simulink model "W01_Base_Map_cs"  (R2019a)
settings: Solver=FixedStepDiscrete  StartTime=0.0  StopTime=40  FixedStep=1/20  RelTol=1e-3
PreLoadFcn:
  | mbxruntime.callbacks.PreLoadFcn(bdroot);
  | check_NUTS_defined
  | model_closed = 0;
  | assignin('base',['model_closed_' bdroot],false);
PostLoadFcn:
  | mbxruntime.callbacks.PostLoadFcn(bdroot);
InitFcn:
  | mbxruntime.callbacks.InitFcn(bdroot);
StartFcn:
  | mbxruntime.callbacks.StartFcn(bdroot);
StopFcn:
  | mbxruntime.callbacks.StopFcn(bdroot);;
  | 
model workspace: external: MAT-File .\W01_Base_Map_cs_hws.mat (data not in the file)
undefined symbols (not defined in the file or in its folder): DiscIntNeverNeededParam, InitImageOutputDir, mbxruntime, tabledata, W01_Base_Map_cs_328ec7e3a8cd5b54, W01_Base_Map_cs_423c72fa17799c7f, W01_Base_Map_cs_514c2dea2cdbe680, W01_Base_Map_cs_51d6e6e467bedba1, W01_Base_Map_cs_563ebd29d1fd6c09, W01_Base_Map_cs_57ea59d0358dab77, W01_Base_Map_cs_669d1acb174df2b9, W01_Base_Map_cs_774a522413284ef7, W01_Base_Map_cs_9538d35a279fbe4e, W01_Base_Map_cs_9f504bb84aebc2fd, W01_Base_Map_cs_a242ed7539861165, W01_Base_Map_cs_ae41b72d7e14f81d, W01_Base_Map_cs_Audi_A8_Sedan_1_Path_pathUniqueID, W01_Base_Map_cs_b5931a786e299506, W01_Base_Map_cs_b7f45a070fa6e639, W01_Base_Map_cs_c02beb48492dde12, W01_Base_Map_cs_c75b75e9f6b035bf, W01_Base_Map_cs_cf83ac8e8b053cbf, W01_Base_Map_cs_Child_RegularAni_1_Path_pathUniqueID, W01_Base_Map_cs_Child_RegularAni_2_Path_pathUniqueID, W01_Base_Map_cs_Citroen_C3_Hatchback_1_Path_pathUniqueID, W01_Base_Map_cs_d4423fcf1c0d6fc4, W01_Base_Map_cs_df133aa86d9852fe, W01_Base_Map_cs_Female_RegularAni_1_Path_pathUniqueID, W01_Base_Map_cs_Male_RegularAni_1_Path_pathUniqueID, W01_Base_Map_cs_Male_RegularAni_2_Path_pathUniqueID
libraries: simulink_extras x41, adeye_lib x15, simulink x10, dspindex x6, PreScanSimulinkLibrary x4, sharedtransform x3, robotcorelib x1, PreScanUsefulBlocks x1
(part 8 of 11)

== system W01_Base_Map_cs/BMW_X5_SUV_1/PointCloudSensor_4_Angles_Demux ==
  In2 : Inport
  Selector : Selector  NumberOfDimensions=2  InputPortWidth=3  IndexOptions=Index vector (dialog),Index vector (dialog)  Indices=-1,offset+1:(offset+hres)  OutputSizes=1,1
  Selector1 : Selector  NumberOfDimensions=2  InputPortWidth=3  IndexOptions=Index vector (dialog),Index vector (dialog)  Indices=-1,(offset+hres+1):(offset+2*hres)  OutputSizes=1,1
  Theta : Outport
  Phi : Outport  Port=2
  wires:
  Selector1/1 -> Phi/1
  Selector/1 -> Theta/1
  In2/1 -> Selector/1, Selector1/1

== system W01_Base_Map_cs/BMW_X5_SUV_1/PointCloudSensor_4_Intensity_Demux ==
  In1 : Inport
  Selector3 : Selector  NumberOfDimensions=2  InputPortWidth=3  IndexOptions=Index vector (dialog),Index vector (dialog)  Indices=-1,offset+1:(offset+hres)  OutputSizes=1,1
  Intensity : Outport
  wires:
  Selector3/1 -> Intensity/1
  In1/1 -> Selector3/1

== system W01_Base_Map_cs/BMW_X5_SUV_1/PointCloudSensor_4_Range_Demux ==
  In1 : Inport
  Selector : Selector  NumberOfDimensions=2  InputPortWidth=3  IndexOptions=Index vector (dialog),Index vector (dialog)  Indices=-1,offset+1:(offset+hres)  OutputSizes=1,1
  Range : Outport
  wires:
  Selector/1 -> Range/1
  In1/1 -> Selector/1

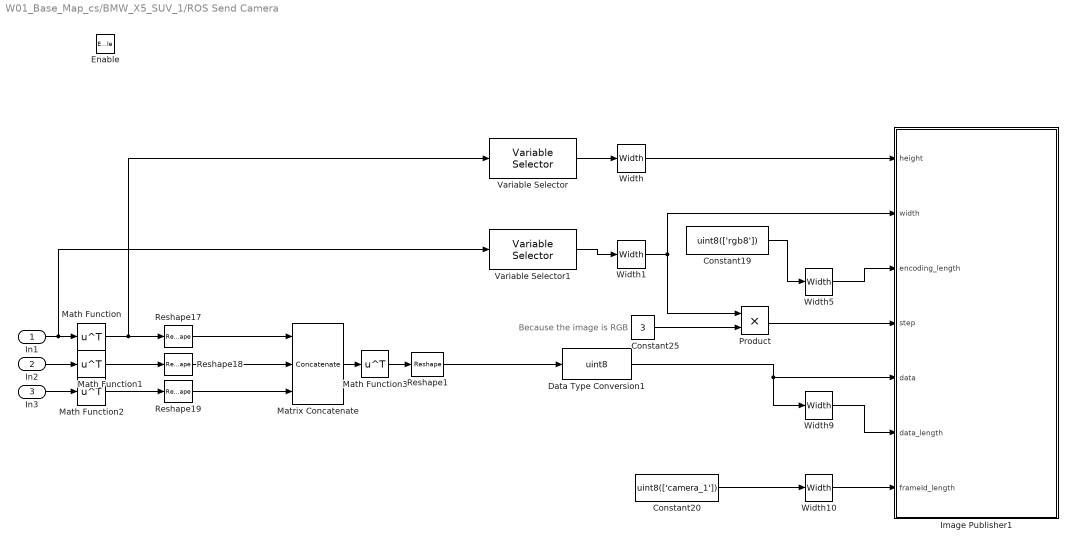
== system W01_Base_Map_cs/BMW_X5_SUV_1/ROS Send Camera ==
  note: Because the image is RGB
  In1 : Inport
  In2 : Inport  Port=2
  In3 : Inport  Port=3
  Enable : EnablePort
  Constant19 : Constant  Value=uint8(['rgb8'])
  Constant20 : Constant  Value=uint8(['camera_1'])
  Constant25 : Constant  Value=3  OutDataTypeStr=Inherit: Inherit via back propagation
  Data Type Conversion1 : DataTypeConversion  OutDataTypeStr=uint8
  Image Publisher1 : Subsystem  mask{topic='/camera_1/image_raw', message_type='sensor_msgs/Image', port=9090, timeout=2, frame_id='camera_1'}
      mask prompts: topic "Topic name"; message_type "Message type"; timeout "Timeout (s)"; frame_id "Frame id (keep '/default' if it's not used)"
  Math Function{,1..3} (4 alike) : Math  Operator=transpose  SaturateOnIntegerOverflow=on
  Matrix Concatenate : Concatenate  NumInputs=3  Mode=Multidimensional array  ConcatenateDimension=2
  Product : Product  OutDataTypeStr=uint32
  Reshape{1,17..19} (4 alike) : Reshape
  Variable Selector : dspindex/Variable Selector  NumInputs=1  rowsOrCols=Rows  IdxMode=Fixed  Elements=[1]  ZerOneIdxMode=One-based  errmode=Clip Index  FillMode=on  FillValues=0
  Variable Selector1 : dspindex/Variable Selector  NumInputs=1  rowsOrCols=Rows  IdxMode=Fixed  Elements=[1]  ZerOneIdxMode=One-based  errmode=Clip Index  FillMode=on  FillValues=0
  Width : Width
  Width1 : Width
  Width10 : Width  DataType=uint32
  Width5 : Width  DataType=uint32
  Width9 : Width  DataType=uint32
  wires:
  Math Function3/1 -> Reshape1/1
  Matrix Concatenate/1 -> Math Function3/1
  In1/1 -> Variable Selector1/1, Math Function/1
  In2/1 -> Math Function1/1
  In3/1 -> Math Function2/1
  Math Function1/1 -> Reshape18/1
  Math Function2/1 -> Reshape19/1
  Reshape17/1 -> Matrix Concatenate/1
  Reshape18/1 -> Matrix Concatenate/2
  Math Function/1 -> Variable Selector/1, Reshape17/1
  Reshape19/1 -> Matrix Concatenate/3
  Constant20/1 -> Width10/1
  Constant25/1 -> Product/2
  Variable Selector1/1 -> Width1/1
  Data Type Conversion1/1 -> Image Publisher1/5(data), Width9/1
  Constant19/1 -> Width5/1
  Variable Selector/1 -> Width/1
  Width1/1 -> Image Publisher1/2(width), Product/1
  Reshape1/1 -> Data Type Conversion1/1
  Width/1 -> Image Publisher1/1(height)
  Product/1 -> Image Publisher1/4(step)
  Width10/1 -> Image Publisher1/7(frameId_length)
  Width5/1 -> Image Publisher1/3(encoding_length)
  Width9/1 -> Image Publisher1/6(data_length)

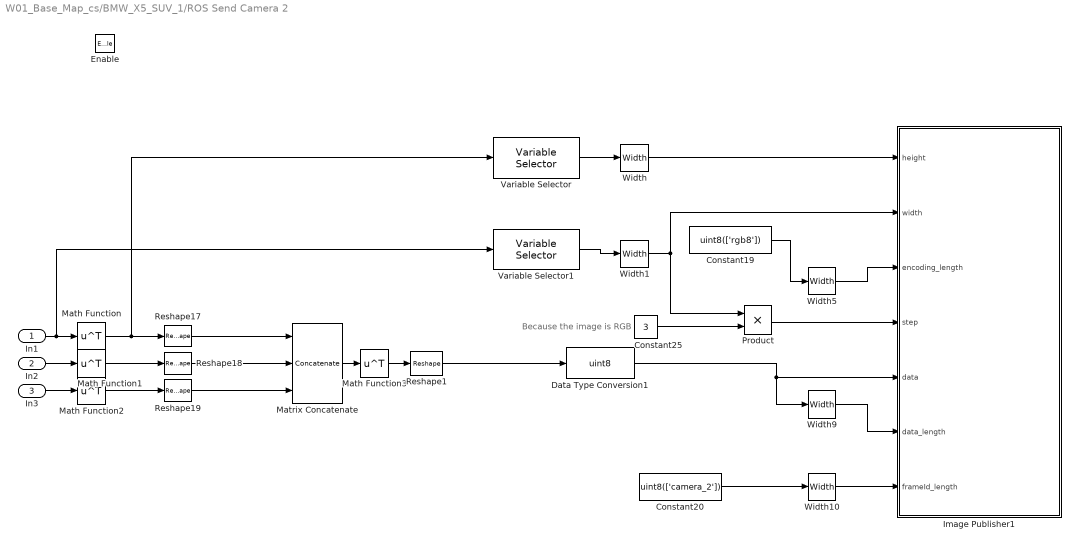
== system W01_Base_Map_cs/BMW_X5_SUV_1/ROS Send Camera 2 ==
  note: Because the image is RGB
  In1 : Inport
  In2 : Inport  Port=2
  In3 : Inport  Port=3
  Enable : EnablePort
  Constant19 : Constant  Value=uint8(['rgb8'])
  Constant20 : Constant  Value=uint8(['camera_2'])
  Constant25 : Constant  Value=3  OutDataTypeStr=Inherit: Inherit via back propagation
  Data Type Conversion1 : DataTypeConversion  OutDataTypeStr=uint8
  Image Publisher1 : Subsystem  mask{topic='/camera_2/image_raw', message_type='sensor_msgs/Image', port=9090, timeout=2, frame_id='camera_2'}
      mask prompts: topic "Topic name"; message_type "Message type"; timeout "Timeout (s)"; frame_id "Frame id (keep '/default' if it's not used)"
  Math Function{,1..3} (4 alike) : Math  Operator=transpose  SaturateOnIntegerOverflow=on
  Matrix Concatenate : Concatenate  NumInputs=3  Mode=Multidimensional array  ConcatenateDimension=2
  Product : Product  OutDataTypeStr=uint32
  Reshape{1,17..19} (4 alike) : Reshape
  Variable Selector : dspindex/Variable Selector  NumInputs=1  rowsOrCols=Rows  IdxMode=Fixed  Elements=[1]  ZerOneIdxMode=One-based  errmode=Clip Index  FillMode=on  FillValues=0
  Variable Selector1 : dspindex/Variable Selector  NumInputs=1  rowsOrCols=Rows  IdxMode=Fixed  Elements=[1]  ZerOneIdxMode=One-based  errmode=Clip Index  FillMode=on  FillValues=0
  Width : Width
  Width1 : Width
  Width10 : Width  DataType=uint32
  Width5 : Width  DataType=uint32
  Width9 : Width  DataType=uint32
  wires:
  Math Function3/1 -> Reshape1/1
  Matrix Concatenate/1 -> Math Function3/1
  In1/1 -> Variable Selector1/1, Math Function/1
  In2/1 -> Math Function1/1
  In3/1 -> Math Function2/1
  Math Function1/1 -> Reshape18/1
  Math Function2/1 -> Reshape19/1
  Reshape17/1 -> Matrix Concatenate/1
  Reshape18/1 -> Matrix Concatenate/2
  Math Function/1 -> Variable Selector/1, Reshape17/1
  Reshape19/1 -> Matrix Concatenate/3
  Width1/1 -> Image Publisher1/2(width), Product/1
  Product/1 -> Image Publisher1/4(step)
  Variable Selector/1 -> Width/1
  Width/1 -> Image Publisher1/1(height)
  Width10/1 -> Image Publisher1/7(frameId_length)
  Data Type Conversion1/1 -> Image Publisher1/5(data), Width9/1
  Reshape1/1 -> Data Type Conversion1/1
  Constant20/1 -> Width10/1
  Variable Selector1/1 -> Width1/1
  Constant25/1 -> Product/2
  Width5/1 -> Image Publisher1/3(encoding_length)
  Width9/1 -> Image Publisher1/6(data_length)
  Constant19/1 -> Width5/1

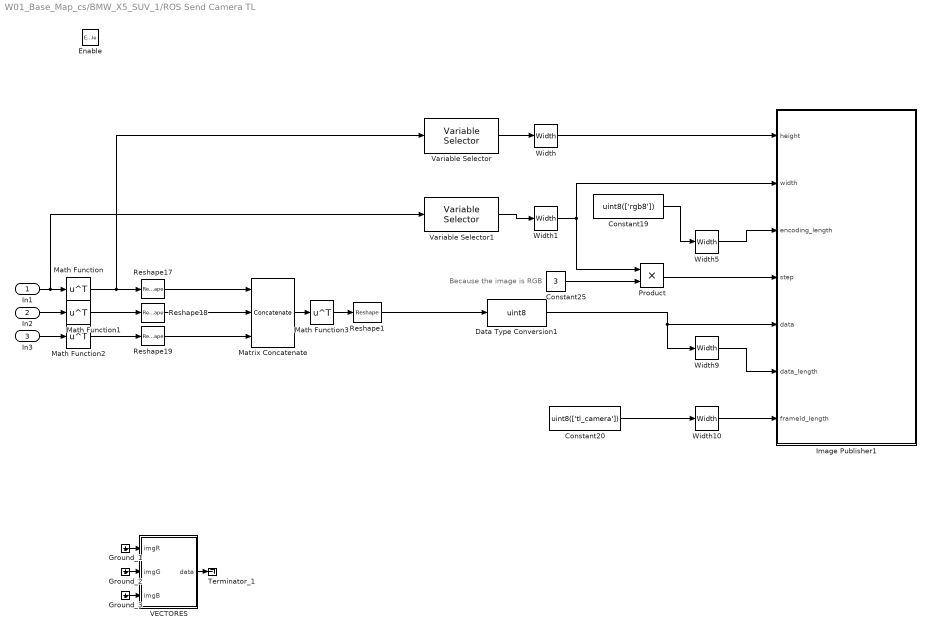
== system W01_Base_Map_cs/BMW_X5_SUV_1/ROS Send Camera TL ==
  note: Because the image is RGB
  In1 : Inport
  In2 : Inport  Port=2
  In3 : Inport  Port=3
  Enable : EnablePort
  Constant19 : Constant  Value=uint8(['rgb8'])
  Constant20 : Constant  Value=uint8(['tl_camera'])
  Constant25 : Constant  Value=3  OutDataTypeStr=Inherit: Inherit via back propagation
  Data Type Conversion1 : DataTypeConversion  OutDataTypeStr=uint8
  Ground_1 : Ground
  Ground_2 : Ground
  Ground_3 : Ground
  Image Publisher1 : Subsystem  mask{topic='/tl/image_raw', message_type='sensor_msgs/Image', port=9090, timeout=2, frame_id='tl_camera'}
      mask prompts: topic "Topic name"; message_type "Message type"; timeout "Timeout (s)"; frame_id "Frame id (keep '/default' if it's not used)"
  Math Function{,1..3} (4 alike) : Math  Operator=transpose  SaturateOnIntegerOverflow=on
  Matrix Concatenate : Concatenate  NumInputs=3  Mode=Multidimensional array  ConcatenateDimension=2
  Product : Product  OutDataTypeStr=uint32
  Reshape{1,17..19} (4 alike) : Reshape
  Terminator_1 : Terminator
  VECTORES : MATLAB Function  TreatAsAtomicUnit=on
  Variable Selector : dspindex/Variable Selector  NumInputs=1  rowsOrCols=Rows  IdxMode=Fixed  Elements=[1]  ZerOneIdxMode=One-based  errmode=Clip Index  FillMode=on  FillValues=0
  Variable Selector1 : dspindex/Variable Selector  NumInputs=1  rowsOrCols=Rows  IdxMode=Fixed  Elements=[1]  ZerOneIdxMode=One-based  errmode=Clip Index  FillMode=on  FillValues=0
  Width : Width
  Width1 : Width
  Width10 : Width  DataType=uint32
  Width5 : Width  DataType=uint32
  Width9 : Width  DataType=uint32
  wires:
  VECTORES/1(data) -> Terminator_1/1
  Ground_3/1 -> VECTORES/3(imgB)
  Ground_2/1 -> VECTORES/2(imgG)
  Ground_1/1 -> VECTORES/1(imgR)
  Math Function3/1 -> Reshape1/1
  Matrix Concatenate/1 -> Math Function3/1
  In1/1 -> Variable Selector1/1, Math Function/1
  In2/1 -> Math Function1/1
  In3/1 -> Math Function2/1
  Math Function1/1 -> Reshape18/1
  Math Function2/1 -> Reshape19/1
  Reshape17/1 -> Matrix Concatenate/1
  Reshape18/1 -> Matrix Concatenate/2
  Math Function/1 -> Variable Selector/1, Reshape17/1
  Reshape19/1 -> Matrix Concatenate/3
  Constant20/1 -> Width10/1
  Constant25/1 -> Product/2
  Variable Selector1/1 -> Width1/1
  Data Type Conversion1/1 -> Image Publisher1/5(data), Width9/1
  Constant19/1 -> Width5/1
  Variable Selector/1 -> Width/1
  Width1/1 -> Image Publisher1/2(width), Product/1
  Reshape1/1 -> Data Type Conversion1/1
  Width/1 -> Image Publisher1/1(height)
  Product/1 -> Image Publisher1/4(step)
  Width10/1 -> Image Publisher1/7(frameId_length)
  Width5/1 -> Image Publisher1/3(encoding_length)
  Width9/1 -> Image Publisher1/6(data_length)

== system W01_Base_Map_cs/BMW_X5_SUV_1/ROS Send Clock ==
  note: Nanoseconds
  In1 : Inport
  Enable : EnablePort
  Clock Publisher : Subsystem  mask{topic='/clock', message_type='rosgraph_msgs/Clock', port=9090, timeout=2}
      mask prompts: topic "Topic name"; message_type "Message type"; timeout "Timeout (s)"
  Constant2 : Constant  Value=1000000000
  Floor : Rounding  Operator=fix
  Product : Product
  Subtract : Sum  Inputs=+-
  wires:
  Constant2/1 -> Product/2
  Product/1 -> Clock Publisher/2(nsecs)
  Subtract/1 -> Product/1
  Floor/1 -> Clock Publisher/1(secs), Subtract/2
  In1/1 -> Floor/1, Subtract/1

== system W01_Base_Map_cs/BMW_X5_SUV_1/ROS Send GNSS ==
  In1 : Inport
  Enable : EnablePort
  Demux : Demux  Outputs=7
  geometry_msgs/Pose : Subsystem  mask{topic='/gnss_pose_simulink', message_type='geometry_msgs/Pose', port=9090, timeout=2}
      mask prompts: topic "Topic name"; message_type "Message type"; timeout "Timeout (s)"
  wires:
  In1/1 -> Demux/1
  Demux/1 -> geometry_msgs/Pose/1(positionX)
  Demux/2 -> geometry_msgs/Pose/2(positionY)
  Demux/3 -> geometry_msgs/Pose/3(positionZ)
  Demux/4 -> geometry_msgs/Pose/4(orientationW)
  Demux/5 -> geometry_msgs/Pose/5(orientationX)
  Demux/6 -> geometry_msgs/Pose/6(orientationY)
  Demux/7 -> geometry_msgs/Pose/7(orientationZ)

== system W01_Base_Map_cs/BMW_X5_SUV_1/ROS Send Goal ==
  In1 : Inport
  In2 : Inport  Port=2
  In3 : Inport  Port=3
  In4 : Inport  Port=4
  In5 : Inport  Port=5
  In6 : Inport  Port=6
  In7 : Inport  Port=7
  Enable : EnablePort
  Add4 : Sum
  Constant8 : Constant  OutDataTypeStr=uint32
  Constant9 : Constant  Value=uint8(['world'])
  Memory1 : Memory  InheritSampleTime=on
  Width4 : Width
  geometry_msgs/PoseStamped : Subsystem  mask{topic='/move_base_simple/goal', message_type='geometry_msgs/PoseStamped', port=9090, timeout=2, frameId='world'}
      mask prompts: topic "Topic name"; message_type "Message type"; timeout "Timeout (s)"
  wires:
  In7/1 -> geometry_msgs/PoseStamped/9(Orientation.z)
  In6/1 -> geometry_msgs/PoseStamped/8(Orientation.y)
  In5/1 -> geometry_msgs/PoseStamped/7(Orientation.x)
  In4/1 -> geometry_msgs/PoseStamped/6(Orientation.w)
  In2/1 -> geometry_msgs/PoseStamped/4(Position.y)
  In1/1 -> geometry_msgs/PoseStamped/3(Position.x)
  Width4/1 -> geometry_msgs/PoseStamped/2(frameId_length)
  Memory1/1 -> Add4/1
  Constant9/1 -> Width4/1
  Constant8/1 -> Add4/2
  Add4/1 -> geometry_msgs/PoseStamped/1(seq), Memory1/1
  In3/1 -> geometry_msgs/PoseStamped/5(Position.z)

== system W01_Base_Map_cs/BMW_X5_SUV_1/ROS Send IMU ==
  In1 : Inport
  In2 : Inport  Port=2
  In3 : Inport  Port=3
  Yaw rate [deg/s] : Inport  Port=4
  Velocity [m/s] : Inport  Port=5
  Enable : EnablePort
  Add5 : Sum
  Constant : Constant  Value=-9.82
  Constant1 : Constant  Value=-1
  Constant24 : Constant  OutDataTypeStr=uint32
  Constant25 : Constant  Value=uint8(['velodyne'])
  Coordinate Transformation Conversion : robotcorelib/Coordinate Transformation Conversion  InputRepresentation=Euler Angles  InputEulerSequence=XYZ  ShowTrVecInputPort=on  OutputRepresentation=Quaternion  OutputEulerSequence=ZYX  ShowTrVecOutputPort=on  SimulateUsing=Interpreted execution
      settings: SourceProductBaseCode=RO
  Degrees to Radians{1..4} (4 alike) : simulink_extras/Transformations/Degrees to Radians
  Demux : Demux
  Derivative : Derivative
  Memory2 : Memory  InheritSampleTime=on
  Product : Product
  Vector Concatenate2 : Concatenate  NumInputs=3
  Width5 : Width
  sensor_msgs/Imu : Subsystem  mask{topic='/imu_raw', message_type='sensor_msgs/Imu', port=9090, timeout=2}
      mask prompts: topic "Topic name"; message_type "Message type"; timeout "Timeout (s)"
  wires:
  Degrees to Radians1/1 -> Vector Concatenate2/1
  Constant24/1 -> Add5/2
  Constant25/1 -> Width5/1
  Width5/1 -> sensor_msgs/Imu/9(frameId_length)
  Add5/1 -> sensor_msgs/Imu/8(seq), Memory2/1
  Memory2/1 -> Add5/1
  Degrees to Radians4/1 -> sensor_msgs/Imu/5(angularZ)
  Derivative/1 -> Product/1
  Degrees to Radians2/1 -> Vector Concatenate2/2
  Demux/2 -> sensor_msgs/Imu/2(orientX)
  Degrees to Radians3/1 -> Vector Concatenate2/3
  Vector Concatenate2/1 -> Coordinate Transformation Conversion/1
  Demux/3 -> sensor_msgs/Imu/3(orientY)
  Coordinate Transformation Conversion/1 -> Demux/1
  Demux/1 -> sensor_msgs/Imu/1(orientW)
  Demux/4 -> sensor_msgs/Imu/4(orientZ)
  Yaw rate [deg/s]/1 -> Degrees to Radians4/1  "Yaw rate [m/s]"
  Velocity [m/s]/1 -> Derivative/1  "Velocity [m/s]"
  Constant/1 -> sensor_msgs/Imu/7(linearAccZ)
  In1/1 -> Degrees to Radians1/1  "Rotational X [deg]"
  In2/1 -> Degrees to Radians2/1  "Rotational Y [deg]"
  In3/1 -> Degrees to Radians3/1  "Rotational Z [deg]"
  Constant1/1 -> Product/2
  Product/1 -> sensor_msgs/Imu/6(linearAccX)

== system W01_Base_Map_cs/BMW_X5_SUV_1/ROS Send Lidar ==
  In1 : Inport
  In5 : Inport  Port=2
  In9 : Inport  Port=3
  In13 : Inport  Port=4
  Enable : EnablePort
  Data Type Conversion2 : DataTypeConversion  OutDataTypeStr=single
  Float32MultiArray Publisher : Subsystem  mask{topic='/points_raw_float32', message_type='std_msgs/Float32MultiArray', port=9090, timeout=2}
      mask prompts: topic "Topic name"; message_type "Message type"; timeout "Timeout (s)"
  Math Function1 : Math  Operator=transpose  SaturateOnIntegerOverflow=on
  Matrix Concatenate5 : Concatenate  NumInputs=4  Mode=Multidimensional array
  Reshape17 : Reshape
  Width5 : Width  DataType=single
  wires:
  Width5/1 -> Float32MultiArray Publisher/2(size)
  Matrix Concatenate5/1 -> Math Function1/1
  Reshape17/1 -> Data Type Conversion2/1
  Data Type Conversion2/1 -> Float32MultiArray Publisher/1(data), Width5/1
  Math Function1/1 -> Reshape17/1
  In1/1 -> Matrix Concatenate5/1
  In5/1 -> Matrix Concatenate5/2
  In9/1 -> Matrix Concatenate5/3
  In13/1 -> Matrix Concatenate5/4

== system W01_Base_Map_cs/BMW_X5_SUV_1/ROS Send Odometry ==
  In1 : Inport
  In2 : Inport  Port=2
  In3 : Inport  Port=3
  Enable : EnablePort
  Add5 : Sum
  Constant{18..21} (4 alike) : Constant  Value=0
  Constant24 : Constant  OutDataTypeStr=uint32
  Constant25 : Constant  Value=uint8(['/base_link'])
  Degrees to Radians3 : simulink_extras/Transformations/Degrees to Radians
  Memory2 : Memory  InheritSampleTime=on
  Width5 : Width
  nav_msgs/Odometry : Subsystem  mask{topic='/vehicle/odom', message_type='nav_msgs/Odometry', port=9090, timeout=2}
      mask prompts: topic "Topic name"; message_type "Message type"; timeout "Timeout (s)"
  wires:
  In2/1 -> nav_msgs/Odometry/4(Velocity)
  Constant21/1 -> nav_msgs/Odometry/8(angularY)
  Constant19/1 -> nav_msgs/Odometry/6(linearZ)
  Constant20/1 -> nav_msgs/Odometry/7(angularX)
  Degrees to Radians3/1 -> nav_msgs/Odometry/9(Yaw rate)
  Constant18/1 -> nav_msgs/Odometry/5(linearY)
  In3/1 -> Degrees to Radians3/1
  Add5/1 -> Memory2/1, nav_msgs/Odometry/1(seq)
  Width5/1 -> nav_msgs/Odometry/2(frameId_length)
  Constant24/1 -> Add5/2
  Memory2/1 -> Add5/1
  Constant25/1 -> Width5/1
  In1/1 -> nav_msgs/Odometry/3(Pose)

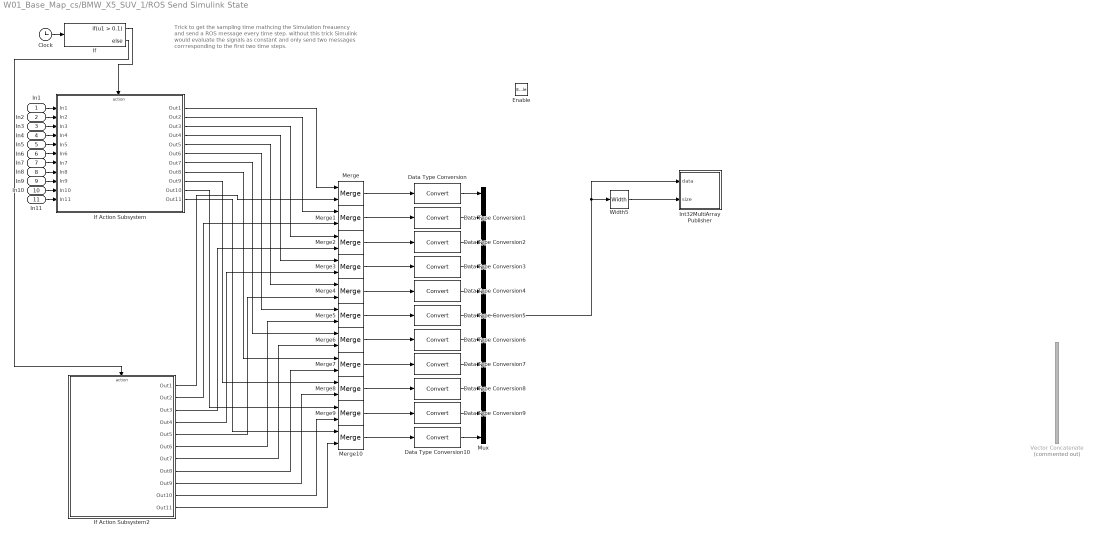
== system W01_Base_Map_cs/BMW_X5_SUV_1/ROS Send Simulink State ==
  note: Trick to get the sampling time mathcing the Simulation freauency and send a ROS message every time step. without this trick Simulink would evaluate the signals as constant and only send two messages corrresponding to the first two time steps.
  In1 : Inport
  In2 : Inport  Port=2
  In3 : Inport  Port=3
  In4 : Inport  Port=4
  In5 : Inport  Port=5
  In6 : Inport  Port=6
  In7 : Inport  Port=7
  In8 : Inport  Port=8
  In9 : Inport  Port=9
  In10 : Inport  Port=10
  In11 : Inport  Port=11
  Enable : EnablePort
  Clock : Clock
  Data Type Conversion{,1..10} (11 alike) : DataTypeConversion
  If : If  IfExpression=u1 > 0.1
  If Action Subsystem : Subsystem  TreatAsAtomicUnit=on
  If Action Subsystem2 : Subsystem  TreatAsAtomicUnit=on
  Int32MultiArray Publisher : Subsystem  mask{topic='/Features_state', message_type='std_msgs/Int32MultiArray', port=9090, timeout=2}
      mask prompts: topic "Topic name"; message_type "Message type"; timeout "Timeout (s)"
  Merge{,1..10} (11 alike) : Merge
  Mux : Mux  Inputs=11
  Vector Concatenate : Concatenate  Commented=on  NumInputs=10
  Width5 : Width
  wires:
  Data Type Conversion10/1 -> Mux/11
  Data Type Conversion9/1 -> Mux/10
  Data Type Conversion8/1 -> Mux/9
  Data Type Conversion7/1 -> Mux/8
  Data Type Conversion6/1 -> Mux/7
  Data Type Conversion5/1 -> Mux/6
  Data Type Conversion4/1 -> Mux/5
  Data Type Conversion3/1 -> Mux/4
  Data Type Conversion2/1 -> Mux/3
  Data Type Conversion1/1 -> Mux/2
  Data Type Conversion/1 -> Mux/1
  If Action Subsystem2/11(Out11) -> Merge10/2
  If Action Subsystem2/10(Out10) -> Merge9/2
  If Action Subsystem2/9(Out9) -> Merge8/2
  If Action Subsystem2/8(Out8) -> Merge7/2
  If Action Subsystem2/7(Out7) -> Merge6/2
  If Action Subsystem2/6(Out6) -> Merge5/2
  If Action Subsystem2/5(Out5) -> Merge4/2
  If Action Subsystem2/4(Out4) -> Merge3/2
  If Action Subsystem2/3(Out3) -> Merge2/2
  If Action Subsystem2/2(Out2) -> Merge1/2
  If Action Subsystem2/1(Out1) -> Merge/2
  If Action Subsystem/11(Out11) -> Merge10/1
  If Action Subsystem/10(Out10) -> Merge9/1
  If Action Subsystem/9(Out9) -> Merge8/1
  If Action Subsystem/8(Out8) -> Merge7/1
  If Action Subsystem/7(Out7) -> Merge6/1
  If Action Subsystem/6(Out6) -> Merge5/1
  If Action Subsystem/5(Out5) -> Merge4/1
  If Action Subsystem/4(Out4) -> Merge3/1
  If Action Subsystem/3(Out3) -> Merge2/1
  If Action Subsystem/2(Out2) -> Merge1/1
  If Action Subsystem/1(Out1) -> Merge/1
  Clock/1 -> If/1
  If/1 -> If Action Subsystem/Action
  If/2 -> If Action Subsystem2/Action
  Merge10/1 -> Data Type Conversion10/1
  Merge9/1 -> Data Type Conversion9/1
  Merge8/1 -> Data Type Conversion8/1
  Merge7/1 -> Data Type Conversion7/1
  Merge6/1 -> Data Type Conversion6/1
  Merge5/1 -> Data Type Conversion5/1
  Merge4/1 -> Data Type Conversion4/1
  Merge3/1 -> Data Type Conversion3/1
  Merge2/1 -> Data Type Conversion2/1
  Merge1/1 -> Data Type Conversion1/1
  Merge/1 -> Data Type Conversion/1
  In1/1 -> If Action Subsystem/1(In1)
  In2/1 -> If Action Subsystem/2(In2)
  In3/1 -> If Action Subsystem/3(In3)
  In4/1 -> If Action Subsystem/4(In4)
  In5/1 -> If Action Subsystem/5(In5)
  In6/1 -> If Action Subsystem/6(In6)
  In7/1 -> If Action Subsystem/7(In7)
  In8/1 -> If Action Subsystem/8(In8)
  In9/1 -> If Action Subsystem/9(In9)
  In10/1 -> If Action Subsystem/10(In10)
  In11/1 -> If Action Subsystem/11(In11)
  Mux/1 -> Int32MultiArray Publisher/1(data), Width5/1
  Width5/1 -> Int32MultiArray Publisher/2(size)

== system W01_Base_Map_cs/BMW_X5_SUV_1/ROS Send Switch Command ==
  In1 : Inport
  Enable : EnablePort
  std_msgs/Int32 Publisher : Subsystem  mask{topic='/switchCommand', message_type='std_msgs/Int32', port=9090, timeout=2}
      mask prompts: topic "Topic name"; message_type "Message type"; timeout "Timeout (s)"
  wires:
  In1/1 -> std_msgs/Int32 Publisher/1(data)

== system W01_Base_Map_cs/BMW_X5_SUV_1/ROS Send Velocity ==
  In1 : Inport
  In2 : Inport  Port=2
  Enable : EnablePort
  Add5 : Sum
  Constant{18..21} (4 alike) : Constant  Value=0
  Constant24 : Constant  OutDataTypeStr=uint32
  Constant25 : Constant  Value=uint8(['/base_link'])
  Degrees to Radians3 : simulink_extras/Transformations/Degrees to Radians
  Memory2 : Memory  InheritSampleTime=on
  Width5 : Width
  geometry_msgs/TwistStamped : Subsystem  mask{topic='/current_velocity', message_type='geometry_msgs/TwistStamped', port=9090, timeout=2}
      mask prompts: topic "Topic name"; message_type "Message type"; timeout "Timeout (s)"
  wires:
  In2/1 -> Degrees to Radians3/1
  In1/1 -> geometry_msgs/TwistStamped/3(linearX)
  Constant21/1 -> geometry_msgs/TwistStamped/7(angularY)
  Constant18/1 -> geometry_msgs/TwistStamped/4(linearY)
  Add5/1 -> geometry_msgs/TwistStamped/1(seq), Memory2/1
  Constant20/1 -> geometry_msgs/TwistStamped/6(angularX)
  Width5/1 -> geometry_msgs/TwistStamped/2(frameId_length)
  Constant24/1 -> Add5/2
  Constant19/1 -> geometry_msgs/TwistStamped/5(linearZ)
  Degrees to Radians3/1 -> geometry_msgs/TwistStamped/8(angularZ)
  Memory2/1 -> Add5/1
  Constant25/1 -> Width5/1

== system W01_Base_Map_cs/BMW_X5_SUV_1/ROS send RCV states ==
  In1 : Inport
  In2 : Inport  Port=2
  In3 : Inport  Port=3
  Bool Publisher : Subsystem  mask{topic='/initial_checks', message_type='std_msgs/Bool', port=9090, timeout=2}
      mask prompts: topic "Topic name"; message_type "Message type"; timeout "Timeout (s)"
  Bool Publisher1 : Subsystem  mask{topic='/activation_request', message_type='std_msgs/Bool', port=9090, timeout=2}
      mask prompts: topic "Topic name"; message_type "Message type"; timeout "Timeout (s)"
  Bool Publisher2 : Subsystem  mask{topic='/fault', message_type='std_msgs/Bool', port=9090, timeout=2}
      mask prompts: topic "Topic name"; message_type "Message type"; timeout "Timeout (s)"
  wires:
  In1/1 -> Bool Publisher/1(data)
  In2/1 -> Bool Publisher1/1(data)
  In3/1 -> Bool Publisher2/1(data)

== system W01_Base_Map_cs/BMW_X5_SUV_1/Radar_1_Demux ==
  Radar : Inport
  Bus Selector1 : BusSelector  OutputSignals=ActiveBeamID[-],Range[m],DopplerVelocity[ms-1],DopplerVelocityX[ms-1],DopplerVelocityY[ms-1],DopplerVelocityZ[ms-1],Theta[deg],Phi[deg],TargetID[-],TargetTypeID[-],EnergyLoss[dB],Alpha[deg],Beta[deg]  OutputAsBus=on
  ScannerSensorLegacyBusConversion : PreScanUsefulBlocks/ScannerSensorLegacyBusConversion  MAXMESSAGES=MAXMESSAGES
  Radar Data : Outport
  wires:
  Bus Selector1/1 -> Radar Data/1
  ScannerSensorLegacyBusConversion/1 -> Bus Selector1/1
  Radar/1 -> ScannerSensorLegacyBusConversion/1

== system W01_Base_Map_cs/BMW_X5_SUV_1/SELF_Demux ==
  SELF : Inport  OutDataTypeStr=Bus: PRESCAN_SELFSENSORDATA
  Bus Selector : BusSelector  OutputSignals=PositionX,PositionY,PositionZ,OrientationRoll,OrientationPitch,OrientationYaw,Velocity,Yaw_rate,Lat,Long,Alt
  Demux2 : Demux  Outputs=3
  Gain : Gain  Gain=180/pi
  Gain1 : Gain  Gain=180/pi
  Vector Concatenate1 : Concatenate  NumInputs=3
  compas converter : Subsystem
  x [m] : Outport
  y [m] : Outport  Port=2
  z [m] : Outport  Port=3
  rotx [deg] : Outport  Port=4
  roty [deg] : Outport  Port=5
  rotz [deg] : Outport  Port=6
  GPS lat [deg] : Outport  Port=7
  GPS long [deg] : Outport  Port=8
  GPS alt [m] : Outport  Port=9
  velocity [m/s] : Outport  Port=10
  heading [deg] : Outport  Port=11
  yaw rate [deg/s] : Outport  Port=12
  wires:
  Bus Selector/11 -> GPS alt [m]/1  "<Alt>"
  Bus Selector/10 -> GPS long [deg]/1  "<Long>"
  Bus Selector/9 -> GPS lat [deg]/1  "<Lat>"
  Bus Selector/8 -> Gain1/1  "<Yaw_rate>"
  Bus Selector/7 -> velocity [m/s]/1  "<Velocity>"
  Bus Selector/6 -> compas converter/1(rotz [rad]), Vector Concatenate1/3  "<OrientationYaw>"
  Bus Selector/5 -> Vector Concatenate1/2  "<OrientationPitch>"
  Bus Selector/4 -> Vector Concatenate1/1  "<OrientationRoll>"
  Vector Concatenate1/1 -> Gain/1
  Bus Selector/3 -> z [m]/1  "<PositionZ>"
  Bus Selector/2 -> y [m]/1  "<PositionY>"
  Bus Selector/1 -> x [m]/1  "<PositionX>"
  SELF/1 -> Bus Selector/1
  Gain/1 -> Demux2/1
  Demux2/1 -> rotx [deg]/1
  Demux2/2 -> roty [deg]/1
  Demux2/3 -> rotz [deg]/1
  compas converter/1(heading [deg]) -> heading [deg]/1
  Gain1/1 -> yaw rate [deg/s]/1

== system W01_Base_Map_cs/BMW_X5_SUV_1/radarDetections ==
  In1 : Inport
  In2 : Inport  Port=2
  In3 : Inport  Port=3
  In4 : Inport  Port=4
  Enable : EnablePort
  Constant : Constant
  Data Type Conversion2 : DataTypeConversion  OutDataTypeStr=single
  Degrees to Radians : simulink_extras/Transformations/Degrees to Radians
  Degrees to Radians1 : simulink_extras/Transformations/Degrees to Radians
  Display3 : Display
  Float32MultiArray Publisher : Subsystem  mask{topic='/radarDetections', message_type='std_msgs/Float32MultiArray', port=9090, timeout=2}
      mask prompts: topic "Topic name"; message_type "Message type"; timeout "Timeout (s)"
  Math Function1 : Math  Operator=transpose  SaturateOnIntegerOverflow=on
  Matrix Concatenate5 : Concatenate  NumInputs=3  Mode=Multidimensional array  ConcatenateDimension=2
  Product : Product
  Product1 : Product
  Product2 : Product
  Relational Operator : RelationalOperator  Operator===  OutDataTypeStr=boolean  RndMeth=Simplest
  Reshape{1..4,17} (5 alike) : Reshape
  Spherical to cartesian : Subsystem
  Width5 : Width  DataType=single
  wires:
  Product1/1 -> Spherical to cartesian/2(In2)
  Math Function1/1 -> Reshape17/1
  Product/1 -> Spherical to cartesian/1(In1)
  Degrees to Radians/1 -> Reshape1/1
  Spherical to cartesian/2(Out2) -> Matrix Concatenate5/2
  Reshape3/1 -> Product2/1
  Degrees to Radians1/1 -> Reshape3/1
  Data Type Conversion2/1 -> Float32MultiArray Publisher/1(data), Width5/1
  Reshape1/1 -> Product1/1
  Reshape17/1 -> Display3/1, Data Type Conversion2/1
  Relational Operator/1 -> Product/2, Product1/2, Product2/2
  In2/1 -> Degrees to Radians/1
  Reshape4/1 -> Relational Operator/1
  In3/1 -> Degrees to Radians1/1
  Reshape2/1 -> Product/1
  Width5/1 -> Float32MultiArray Publisher/2(size)
  Spherical to cartesian/1(Out1) -> Matrix Concatenate5/1
  In1/1 -> Reshape2/1
  Matrix Concatenate5/1 -> Math Function1/1
  Product2/1 -> Spherical to cartesian/3(In3)
  In4/1 -> Reshape4/1
  Spherical to cartesian/3(Out3) -> Matrix Concatenate5/3
  Constant/1 -> Relational Operator/2

== system W01_Base_Map_cs/Child_RegularAni_1/Animation ==
  In1 : Inport
  Bus Creator : BusCreator  Inputs=2  OutDataTypeStr=Bus: PRESCAN_ANIMACTUATORDATA  NonVirtualBus=on
  Bus Selector : BusSelector  OutputSignals=VelocityX,VelocityY,VelocityZ
  Data Type Conversion : DataTypeConversion  OutDataTypeStr=int32
  Mux : Mux  Inputs=3
  Product : Product  RndMeth=Zero
  RunningScale : Constant  Value=RunningScale
  Switch : Switch  Threshold=2
  WalkingScale : Constant  Value=WalkingScale
  animation mode : Subsystem
  elapsed track : Subsystem
  Out1 : Outport
  wires:
  Switch/1 -> Product/1
  WalkingScale/1 -> Switch/3
  RunningScale/1 -> Switch/1
  elapsed track/1(s) -> Product/2  "Time"
  Product/1 -> Bus Creator/2  "Time"
  Mux/1 -> elapsed track/1(vel), animation mode/1(vel)
  Bus Selector/1 -> Mux/1  "<VelocityX>"
  Bus Selector/2 -> Mux/2  "<VelocityY>"
  Bus Selector/3 -> Mux/3  "<VelocityZ>"
  animation mode/1(mode) -> Switch/2, Data Type Conversion/1
  In1/1 -> Bus Selector/1
  Bus Creator/1 -> Out1/1
  Data Type Conversion/1 -> Bus Creator/1  "Index"

== system W01_Base_Map_cs/Child_RegularAni_1/SELF_Demux ==
  SELF : Inport  OutDataTypeStr=Bus: PRESCAN_SELFSENSORDATA
  Bus Selector : BusSelector  OutputSignals=PositionX,PositionY,PositionZ,OrientationRoll,OrientationPitch,OrientationYaw,Velocity,Yaw_rate,Lat,Long,Alt
  Demux2 : Demux  Outputs=3
  Gain : Gain  Gain=180/pi
  Gain1 : Gain  Gain=180/pi
  Vector Concatenate1 : Concatenate  NumInputs=3
  compas converter : Subsystem
  x [m] : Outport
  y [m] : Outport  Port=2
  z [m] : Outport  Port=3
  rotx [deg] : Outport  Port=4
  roty [deg] : Outport  Port=5
  rotz [deg] : Outport  Port=6
  GPS lat [deg] : Outport  Port=7
  GPS long [deg] : Outport  Port=8
  GPS alt [m] : Outport  Port=9
  velocity [m/s] : Outport  Port=10
  heading [deg] : Outport  Port=11
  yaw rate [deg/s] : Outport  Port=12
  wires:
  Bus Selector/11 -> GPS alt [m]/1  "<Alt>"
  Bus Selector/10 -> GPS long [deg]/1  "<Long>"
  Bus Selector/9 -> GPS lat [deg]/1  "<Lat>"
  Bus Selector/8 -> Gain1/1  "<Yaw_rate>"
  Bus Selector/7 -> velocity [m/s]/1  "<Velocity>"
  Bus Selector/6 -> compas converter/1(rotz [rad]), Vector Concatenate1/3  "<OrientationYaw>"
  Bus Selector/5 -> Vector Concatenate1/2  "<OrientationPitch>"
  Bus Selector/4 -> Vector Concatenate1/1  "<OrientationRoll>"
  Vector Concatenate1/1 -> Gain/1
  Bus Selector/3 -> z [m]/1  "<PositionZ>"
  Bus Selector/2 -> y [m]/1  "<PositionY>"
  Bus Selector/1 -> x [m]/1  "<PositionX>"
  SELF/1 -> Bus Selector/1
  Gain/1 -> Demux2/1
  Demux2/1 -> rotx [deg]/1
  Demux2/2 -> roty [deg]/1
  Demux2/3 -> rotz [deg]/1
  compas converter/1(heading [deg]) -> heading [deg]/1
  Gain1/1 -> yaw rate [deg/s]/1

== system W01_Base_Map_cs/Child_RegularAni_1/VISUColorRegion_Lower_Body_Mux ==
  RGB [-,-,-] : Inport
  Bus Creator : BusCreator  Inputs=4  OutDataTypeStr=Bus: PRESCAN_COLOR_DATA  NonVirtualBus=on
  Constant : Constant  Value=255  OutDataTypeStr=uint8
  Data Type Conversion : DataTypeConversion  OutDataTypeStr=uint8
  Data Type Conversion1 : DataTypeConversion  OutDataTypeStr=uint8
  Data Type Conversion2 : DataTypeConversion  OutDataTypeStr=uint8
  Demux : Demux  Outputs=3
  ColorRegion : Outport  OutDataTypeStr=Bus: PRESCAN_COLOR_DATA  PortDimensions=1
  wires:
  Constant/1 -> Bus Creator/4  "A"
  Data Type Conversion2/1 -> Bus Creator/3  "B"
  Data Type Conversion1/1 -> Bus Creator/2  "G"
  Data Type Conversion/1 -> Bus Creator/1  "R"
  Demux/3 -> Data Type Conversion2/1  "B"
  Demux/2 -> Data Type Conversion1/1  "G"
  Demux/1 -> Data Type Conversion/1  "R"
  RGB [-,-,-]/1 -> Demux/1
  Bus Creator/1 -> ColorRegion/1

== system W01_Base_Map_cs/Child_RegularAni_1/VISUColorRegion_Shoes_Mux ==
  RGB [-,-,-] : Inport
  Bus Creator : BusCreator  Inputs=4  OutDataTypeStr=Bus: PRESCAN_COLOR_DATA  NonVirtualBus=on
  Constant : Constant  Value=255  OutDataTypeStr=uint8
  Data Type Conversion : DataTypeConversion  OutDataTypeStr=uint8
  Data Type Conversion1 : DataTypeConversion  OutDataTypeStr=uint8
  Data Type Conversion2 : DataTypeConversion  OutDataTypeStr=uint8
  Demux : Demux  Outputs=3
  ColorRegion : Outport  OutDataTypeStr=Bus: PRESCAN_COLOR_DATA  PortDimensions=1
  wires:
  Constant/1 -> Bus Creator/4  "A"
  Data Type Conversion2/1 -> Bus Creator/3  "B"
  Data Type Conversion1/1 -> Bus Creator/2  "G"
  Data Type Conversion/1 -> Bus Creator/1  "R"
  Demux/3 -> Data Type Conversion2/1  "B"
  Demux/2 -> Data Type Conversion1/1  "G"
  Demux/1 -> Data Type Conversion/1  "R"
  RGB [-,-,-]/1 -> Demux/1
  Bus Creator/1 -> ColorRegion/1

== system W01_Base_Map_cs/Child_RegularAni_1/VISUColorRegion_Upper_Body_Mux ==
  RGB [-,-,-] : Inport
  Bus Creator : BusCreator  Inputs=4  OutDataTypeStr=Bus: PRESCAN_COLOR_DATA  NonVirtualBus=on
  Constant : Constant  Value=255  OutDataTypeStr=uint8
  Data Type Conversion : DataTypeConversion  OutDataTypeStr=uint8
  Data Type Conversion1 : DataTypeConversion  OutDataTypeStr=uint8
  Data Type Conversion2 : DataTypeConversion  OutDataTypeStr=uint8
  Demux : Demux  Outputs=3
  ColorRegion : Outport  OutDataTypeStr=Bus: PRESCAN_COLOR_DATA  PortDimensions=1
  wires:
  Constant/1 -> Bus Creator/4  "A"
  Data Type Conversion2/1 -> Bus Creator/3  "B"
  Data Type Conversion1/1 -> Bus Creator/2  "G"
  Data Type Conversion/1 -> Bus Creator/1  "R"
  Demux/3 -> Data Type Conversion2/1  "B"
  Demux/2 -> Data Type Conversion1/1  "G"
  Demux/1 -> Data Type Conversion/1  "R"
  RGB [-,-,-]/1 -> Demux/1
  Bus Creator/1 -> ColorRegion/1

== system W01_Base_Map_cs/Child_RegularAni_2/Animation ==
  In1 : Inport
  Bus Creator : BusCreator  Inputs=2  OutDataTypeStr=Bus: PRESCAN_ANIMACTUATORDATA  NonVirtualBus=on
  Bus Selector : BusSelector  OutputSignals=VelocityX,VelocityY,VelocityZ
  Data Type Conversion : DataTypeConversion  OutDataTypeStr=int32
  Mux : Mux  Inputs=3
  Product : Product  RndMeth=Zero
  RunningScale : Constant  Value=RunningScale
  Switch : Switch  Threshold=2
  WalkingScale : Constant  Value=WalkingScale
  animation mode : Subsystem
  elapsed track : Subsystem
  Out1 : Outport
  wires:
  Switch/1 -> Product/1
  WalkingScale/1 -> Switch/3
  RunningScale/1 -> Switch/1
  elapsed track/1(s) -> Product/2  "Time"
  Product/1 -> Bus Creator/2  "Time"
  Mux/1 -> elapsed track/1(vel), animation mode/1(vel)
  Bus Selector/1 -> Mux/1  "<VelocityX>"
  Bus Selector/2 -> Mux/2  "<VelocityY>"
  Bus Selector/3 -> Mux/3  "<VelocityZ>"
  animation mode/1(mode) -> Switch/2, Data Type Conversion/1
  In1/1 -> Bus Selector/1
  Bus Creator/1 -> Out1/1
  Data Type Conversion/1 -> Bus Creator/1  "Index"

== system W01_Base_Map_cs/Child_RegularAni_2/SELF_Demux ==
  SELF : Inport  OutDataTypeStr=Bus: PRESCAN_SELFSENSORDATA
  Bus Selector : BusSelector  OutputSignals=PositionX,PositionY,PositionZ,OrientationRoll,OrientationPitch,OrientationYaw,Velocity,Yaw_rate,Lat,Long,Alt
  Demux2 : Demux  Outputs=3
  Gain : Gain  Gain=180/pi
  Gain1 : Gain  Gain=180/pi
  Vector Concatenate1 : Concatenate  NumInputs=3
  compas converter : Subsystem
  x [m] : Outport
  y [m] : Outport  Port=2
  z [m] : Outport  Port=3
  rotx [deg] : Outport  Port=4
  roty [deg] : Outport  Port=5
  rotz [deg] : Outport  Port=6
  GPS lat [deg] : Outport  Port=7
  GPS long [deg] : Outport  Port=8
  GPS alt [m] : Outport  Port=9
  velocity [m/s] : Outport  Port=10
  heading [deg] : Outport  Port=11
  yaw rate [deg/s] : Outport  Port=12
  wires:
  Bus Selector/11 -> GPS alt [m]/1  "<Alt>"
  Bus Selector/10 -> GPS long [deg]/1  "<Long>"
  Bus Selector/9 -> GPS lat [deg]/1  "<Lat>"
  Bus Selector/8 -> Gain1/1  "<Yaw_rate>"
  Bus Selector/7 -> velocity [m/s]/1  "<Velocity>"
  Bus Selector/6 -> compas converter/1(rotz [rad]), Vector Concatenate1/3  "<OrientationYaw>"
  Bus Selector/5 -> Vector Concatenate1/2  "<OrientationPitch>"
  Bus Selector/4 -> Vector Concatenate1/1  "<OrientationRoll>"
  Vector Concatenate1/1 -> Gain/1
  Bus Selector/3 -> z [m]/1  "<PositionZ>"
  Bus Selector/2 -> y [m]/1  "<PositionY>"
  Bus Selector/1 -> x [m]/1  "<PositionX>"
  SELF/1 -> Bus Selector/1
  Gain/1 -> Demux2/1
  Demux2/1 -> rotx [deg]/1
  Demux2/2 -> roty [deg]/1
  Demux2/3 -> rotz [deg]/1
  compas converter/1(heading [deg]) -> heading [deg]/1
  Gain1/1 -> yaw rate [deg/s]/1

== system W01_Base_Map_cs/Child_RegularAni_2/VISUColorRegion_Lower_Body_Mux ==
  RGB [-,-,-] : Inport
  Bus Creator : BusCreator  Inputs=4  OutDataTypeStr=Bus: PRESCAN_COLOR_DATA  NonVirtualBus=on
  Constant : Constant  Value=255  OutDataTypeStr=uint8
  Data Type Conversion : DataTypeConversion  OutDataTypeStr=uint8
  Data Type Conversion1 : DataTypeConversion  OutDataTypeStr=uint8
  Data Type Conversion2 : DataTypeConversion  OutDataTypeStr=uint8
  Demux : Demux  Outputs=3
  ColorRegion : Outport  OutDataTypeStr=Bus: PRESCAN_COLOR_DATA  PortDimensions=1
  wires:
  Constant/1 -> Bus Creator/4  "A"
  Data Type Conversion2/1 -> Bus Creator/3  "B"
  Data Type Conversion1/1 -> Bus Creator/2  "G"
  Data Type Conversion/1 -> Bus Creator/1  "R"
  Demux/3 -> Data Type Conversion2/1  "B"
  Demux/2 -> Data Type Conversion1/1  "G"
  Demux/1 -> Data Type Conversion/1  "R"
  RGB [-,-,-]/1 -> Demux/1
  Bus Creator/1 -> ColorRegion/1

== system W01_Base_Map_cs/Child_RegularAni_2/VISUColorRegion_Shoes_Mux ==
  RGB [-,-,-] : Inport
  Bus Creator : BusCreator  Inputs=4  OutDataTypeStr=Bus: PRESCAN_COLOR_DATA  NonVirtualBus=on
  Constant : Constant  Value=255  OutDataTypeStr=uint8
  Data Type Conversion : DataTypeConversion  OutDataTypeStr=uint8
  Data Type Conversion1 : DataTypeConversion  OutDataTypeStr=uint8
  Data Type Conversion2 : DataTypeConversion  OutDataTypeStr=uint8
  Demux : Demux  Outputs=3
  ColorRegion : Outport  OutDataTypeStr=Bus: PRESCAN_COLOR_DATA  PortDimensions=1
  wires:
  Constant/1 -> Bus Creator/4  "A"
  Data Type Conversion2/1 -> Bus Creator/3  "B"
  Data Type Conversion1/1 -> Bus Creator/2  "G"
  Data Type Conversion/1 -> Bus Creator/1  "R"
  Demux/3 -> Data Type Conversion2/1  "B"
  Demux/2 -> Data Type Conversion1/1  "G"
  Demux/1 -> Data Type Conversion/1  "R"
  RGB [-,-,-]/1 -> Demux/1
  Bus Creator/1 -> ColorRegion/1

== system W01_Base_Map_cs/Child_RegularAni_2/VISUColorRegion_Upper_Body_Mux ==
  RGB [-,-,-] : Inport
  Bus Creator : BusCreator  Inputs=4  OutDataTypeStr=Bus: PRESCAN_COLOR_DATA  NonVirtualBus=on
  Constant : Constant  Value=255  OutDataTypeStr=uint8
  Data Type Conversion : DataTypeConversion  OutDataTypeStr=uint8
  Data Type Conversion1 : DataTypeConversion  OutDataTypeStr=uint8
  Data Type Conversion2 : DataTypeConversion  OutDataTypeStr=uint8
  Demux : Demux  Outputs=3
  ColorRegion : Outport  OutDataTypeStr=Bus: PRESCAN_COLOR_DATA  PortDimensions=1
  wires:
  Constant/1 -> Bus Creator/4  "A"
  Data Type Conversion2/1 -> Bus Creator/3  "B"
  Data Type Conversion1/1 -> Bus Creator/2  "G"
  Data Type Conversion/1 -> Bus Creator/1  "R"
  Demux/3 -> Data Type Conversion2/1  "B"
  Demux/2 -> Data Type Conversion1/1  "G"
  Demux/1 -> Data Type Conversion/1  "R"
  RGB [-,-,-]/1 -> Demux/1
  Bus Creator/1 -> ColorRegion/1

== system W01_Base_Map_cs/Citroen_C3_Hatchback_1/Car_Pos_and_Orient ==
  In1 : Inport
  In2 : Inport  Port=2
  In3 : Inport  Port=3
  In4 : Inport  Port=4
  In5 : Inport  Port=5
  In6 : Inport  Port=6
  Data Type Conversion : DataTypeConversion
  Data Type Conversion1 : DataTypeConversion
  Data Type Conversion2 : DataTypeConversion
  Degrees to Radians1 : simulink_extras/Transformations/Degrees to Radians
  Degrees to Radians2 : simulink_extras/Transformations/Degrees to Radians
  Degrees to Radians5 : simulink_extras/Transformations/Degrees to Radians
  Mux : Mux
  Rotation Angles to Quaternions : sharedtransform/Rotation Angles to Quaternions  rotationOrder=XYZ  aMode=aMode
      settings: SourceProductName=Aerospace Blockset  SourceProductBaseCode=AE
  Vector Concatenate2 : Concatenate  NumInputs=3
  Out1 : Outport
  wires:
  Degrees to Radians1/1 -> Vector Concatenate2/2
  Degrees to Radians5/1 -> Vector Concatenate2/1
  Vector Concatenate2/1 -> Rotation Angles to Quaternions/1
  Degrees to Radians2/1 -> Vector Concatenate2/3
  In1/1 -> Data Type Conversion/1
  In2/1 -> Data Type Conversion1/1
  In3/1 -> Data Type Conversion2/1
  In4/1 -> Degrees to Radians5/1
  In5/1 -> Degrees to Radians1/1
  In6/1 -> Degrees to Radians2/1
  Data Type Conversion/1 -> Mux/1
  Data Type Conversion1/1 -> Mux/2
  Data Type Conversion2/1 -> Mux/3
  Rotation Angles to Quaternions/1 -> Mux/4
  Mux/1 -> Out1/1

== system W01_Base_Map_cs/Citroen_C3_Hatchback_1/SELF_Demux ==
  SELF : Inport  OutDataTypeStr=Bus: PRESCAN_SELFSENSORDATA
  Bus Selector : BusSelector  OutputSignals=PositionX,PositionY,PositionZ,OrientationRoll,OrientationPitch,OrientationYaw,Velocity,Yaw_rate,Lat,Long,Alt
  Demux2 : Demux  Outputs=3
  Gain : Gain  Gain=180/pi
  Gain1 : Gain  Gain=180/pi
  Vector Concatenate1 : Concatenate  NumInputs=3
  compas converter : Subsystem
  x [m] : Outport
  y [m] : Outport  Port=2
  z [m] : Outport  Port=3
  rotx [deg] : Outport  Port=4
  roty [deg] : Outport  Port=5
  rotz [deg] : Outport  Port=6
  GPS lat [deg] : Outport  Port=7
  GPS long [deg] : Outport  Port=8
  GPS alt [m] : Outport  Port=9
  velocity [m/s] : Outport  Port=10
  heading [deg] : Outport  Port=11
  yaw rate [deg/s] : Outport  Port=12
  wires:
  Bus Selector/11 -> GPS alt [m]/1  "<Alt>"
  Bus Selector/10 -> GPS long [deg]/1  "<Long>"
  Bus Selector/9 -> GPS lat [deg]/1  "<Lat>"
  Bus Selector/8 -> Gain1/1  "<Yaw_rate>"
  Bus Selector/7 -> velocity [m/s]/1  "<Velocity>"
  Bus Selector/6 -> compas converter/1(rotz [rad]), Vector Concatenate1/3  "<OrientationYaw>"
  Bus Selector/5 -> Vector Concatenate1/2  "<OrientationPitch>"
  Bus Selector/4 -> Vector Concatenate1/1  "<OrientationRoll>"
  Vector Concatenate1/1 -> Gain/1
  Bus Selector/3 -> z [m]/1  "<PositionZ>"
  Bus Selector/2 -> y [m]/1  "<PositionY>"
  Bus Selector/1 -> x [m]/1  "<PositionX>"
  SELF/1 -> Bus Selector/1
  Gain/1 -> Demux2/1
  Demux2/1 -> rotx [deg]/1
  Demux2/2 -> roty [deg]/1
  Demux2/3 -> rotz [deg]/1
  compas converter/1(heading [deg]) -> heading [deg]/1
  Gain1/1 -> yaw rate [deg/s]/1

== system W01_Base_Map_cs/Female_RegularAni_1/Animation ==
  In1 : Inport
  Bus Creator : BusCreator  Inputs=2  OutDataTypeStr=Bus: PRESCAN_ANIMACTUATORDATA  NonVirtualBus=on
  Bus Selector : BusSelector  OutputSignals=VelocityX,VelocityY,VelocityZ
  Data Type Conversion : DataTypeConversion  OutDataTypeStr=int32
  Mux : Mux  Inputs=3
  Product : Product  RndMeth=Zero
  RunningScale : Constant  Value=RunningScale
  Switch : Switch  Threshold=2
  WalkingScale : Constant  Value=WalkingScale
  animation mode : Subsystem
  elapsed track : Subsystem
  Out1 : Outport
  wires:
  Switch/1 -> Product/1
  WalkingScale/1 -> Switch/3
  RunningScale/1 -> Switch/1
  elapsed track/1(s) -> Product/2  "Time"
  Product/1 -> Bus Creator/2  "Time"
  Mux/1 -> elapsed track/1(vel), animation mode/1(vel)
  Bus Selector/1 -> Mux/1  "<VelocityX>"
  Bus Selector/2 -> Mux/2  "<VelocityY>"
  Bus Selector/3 -> Mux/3  "<VelocityZ>"
  animation mode/1(mode) -> Switch/2, Data Type Conversion/1
  In1/1 -> Bus Selector/1
  Bus Creator/1 -> Out1/1
  Data Type Conversion/1 -> Bus Creator/1  "Index"

== system W01_Base_Map_cs/Female_RegularAni_1/SELF_Demux ==
  SELF : Inport  OutDataTypeStr=Bus: PRESCAN_SELFSENSORDATA
  Bus Selector : BusSelector  OutputSignals=PositionX,PositionY,PositionZ,OrientationRoll,OrientationPitch,OrientationYaw,Velocity,Yaw_rate,Lat,Long,Alt
  Demux2 : Demux  Outputs=3
  Gain : Gain  Gain=180/pi
  Gain1 : Gain  Gain=180/pi
  Vector Concatenate1 : Concatenate  NumInputs=3
  compas converter : Subsystem
  x [m] : Outport
  y [m] : Outport  Port=2
  z [m] : Outport  Port=3
  rotx [deg] : Outport  Port=4
  roty [deg] : Outport  Port=5
  rotz [deg] : Outport  Port=6
  GPS lat [deg] : Outport  Port=7
  GPS long [deg] : Outport  Port=8
  GPS alt [m] : Outport  Port=9
  velocity [m/s] : Outport  Port=10
  heading [deg] : Outport  Port=11
  yaw rate [deg/s] : Outport  Port=12
  wires:
  Bus Selector/11 -> GPS alt [m]/1  "<Alt>"
  Bus Selector/10 -> GPS long [deg]/1  "<Long>"
  Bus Selector/9 -> GPS lat [deg]/1  "<Lat>"
  Bus Selector/8 -> Gain1/1  "<Yaw_rate>"
  Bus Selector/7 -> velocity [m/s]/1  "<Velocity>"
  Bus Selector/6 -> compas converter/1(rotz [rad]), Vector Concatenate1/3  "<OrientationYaw>"
  Bus Selector/5 -> Vector Concatenate1/2  "<OrientationPitch>"
  Bus Selector/4 -> Vector Concatenate1/1  "<OrientationRoll>"
  Vector Concatenate1/1 -> Gain/1
  Bus Selector/3 -> z [m]/1  "<PositionZ>"
  Bus Selector/2 -> y [m]/1  "<PositionY>"
  Bus Selector/1 -> x [m]/1  "<PositionX>"
  SELF/1 -> Bus Selector/1
  Gain/1 -> Demux2/1
  Demux2/1 -> rotx [deg]/1
  Demux2/2 -> roty [deg]/1
  Demux2/3 -> rotz [deg]/1
  compas converter/1(heading [deg]) -> heading [deg]/1
  Gain1/1 -> yaw rate [deg/s]/1

== system W01_Base_Map_cs/Female_RegularAni_1/VISUColorRegion_Lower_Body_Mux ==
  RGB [-,-,-] : Inport
  Bus Creator : BusCreator  Inputs=4  OutDataTypeStr=Bus: PRESCAN_COLOR_DATA  NonVirtualBus=on
  Constant : Constant  Value=255  OutDataTypeStr=uint8
  Data Type Conversion : DataTypeConversion  OutDataTypeStr=uint8
  Data Type Conversion1 : DataTypeConversion  OutDataTypeStr=uint8
  Data Type Conversion2 : DataTypeConversion  OutDataTypeStr=uint8
  Demux : Demux  Outputs=3
  ColorRegion : Outport  OutDataTypeStr=Bus: PRESCAN_COLOR_DATA  PortDimensions=1
  wires:
  Constant/1 -> Bus Creator/4  "A"
  Data Type Conversion2/1 -> Bus Creator/3  "B"
  Data Type Conversion1/1 -> Bus Creator/2  "G"
  Data Type Conversion/1 -> Bus Creator/1  "R"
  Demux/3 -> Data Type Conversion2/1  "B"
  Demux/2 -> Data Type Conversion1/1  "G"
  Demux/1 -> Data Type Conversion/1  "R"
  RGB [-,-,-]/1 -> Demux/1
  Bus Creator/1 -> ColorRegion/1

== system W01_Base_Map_cs/Female_RegularAni_1/VISUColorRegion_Shoes_Mux ==
  RGB [-,-,-] : Inport
  Bus Creator : BusCreator  Inputs=4  OutDataTypeStr=Bus: PRESCAN_COLOR_DATA  NonVirtualBus=on
  Constant : Constant  Value=255  OutDataTypeStr=uint8
  Data Type Conversion : DataTypeConversion  OutDataTypeStr=uint8
  Data Type Conversion1 : DataTypeConversion  OutDataTypeStr=uint8
  Data Type Conversion2 : DataTypeConversion  OutDataTypeStr=uint8
  Demux : Demux  Outputs=3
  ColorRegion : Outport  OutDataTypeStr=Bus: PRESCAN_COLOR_DATA  PortDimensions=1
  wires:
  Constant/1 -> Bus Creator/4  "A"
  Data Type Conversion2/1 -> Bus Creator/3  "B"
  Data Type Conversion1/1 -> Bus Creator/2  "G"
  Data Type Conversion/1 -> Bus Creator/1  "R"
  Demux/3 -> Data Type Conversion2/1  "B"
  Demux/2 -> Data Type Conversion1/1  "G"
  Demux/1 -> Data Type Conversion/1  "R"
  RGB [-,-,-]/1 -> Demux/1
  Bus Creator/1 -> ColorRegion/1

== system W01_Base_Map_cs/Female_RegularAni_1/VISUColorRegion_Upper_Body_Mux ==
  RGB [-,-,-] : Inport
  Bus Creator : BusCreator  Inputs=4  OutDataTypeStr=Bus: PRESCAN_COLOR_DATA  NonVirtualBus=on
  Constant : Constant  Value=255  OutDataTypeStr=uint8
  Data Type Conversion : DataTypeConversion  OutDataTypeStr=uint8
  Data Type Conversion1 : DataTypeConversion  OutDataTypeStr=uint8
  Data Type Conversion2 : DataTypeConversion  OutDataTypeStr=uint8
  Demux : Demux  Outputs=3
  ColorRegion : Outport  OutDataTypeStr=Bus: PRESCAN_COLOR_DATA  PortDimensions=1
  wires:
  Constant/1 -> Bus Creator/4  "A"
  Data Type Conversion2/1 -> Bus Creator/3  "B"
  Data Type Conversion1/1 -> Bus Creator/2  "G"
  Data Type Conversion/1 -> Bus Creator/1  "R"
  Demux/3 -> Data Type Conversion2/1  "B"
  Demux/2 -> Data Type Conversion1/1  "G"
  Demux/1 -> Data Type Conversion/1  "R"
  RGB [-,-,-]/1 -> Demux/1
  Bus Creator/1 -> ColorRegion/1
